simulink model "PPTS_pmsm"  (R2020b)
settings: Solver=ode3  StartTime=0.0  StopTime=10.0  FixedStep=0.0001  RelTol=0.0001
values from neighbouring files (symbols this model uses):
  a = 0.3    [initial_parameters_PPTS.m]
  a11 = 48    [initial_parameters_PPTS.m]
  a12 = 48    [initial_parameters_PPTS.m]
  a21 = 13    [initial_parameters_PPTS.m]
  a22 = 13    [initial_parameters_PPTS.m]
  B = 2e-3    (= 0.002)    [initial_parameters_PPTS.m]
  f = 1    [initial_parameters_PPTS.m]
  J = 8e-4    (= 0.0008)    [initial_parameters_PPTS.m]
  k1 = 240    [initial_parameters_PPTS.m]
  K1 = 220    [initial_parameters_PPTS.m]
  k2 = 240    [initial_parameters_PPTS.m]
  K2 = 220    [initial_parameters_PPTS.m]
  k3 = 240    [initial_parameters_PPTS.m]
  K3 = 220    [initial_parameters_PPTS.m]
  k4 = 240    [initial_parameters_PPTS.m]
  K4 = 220    [initial_parameters_PPTS.m]
  L = 0.1875    [initial_parameters_PPTS.m]
  n1 = 0.9    [initial_parameters_PPTS.m]
  n2 = 0.7    [initial_parameters_PPTS.m]
  P = 2    [initial_parameters_PPTS.m]
  psi_f = 0.945    [initial_parameters_PPTS.m]
  R = 12.5    [initial_parameters_PPTS.m]
  rh0 = 0.8    [initial_parameters_PPTS.m]
  rh0c = 0.9    [initial_parameters_PPTS.m]
  rho0 = 10.6    [initial_parameters_PPTS.m]
  rho01 = 0.6    [initial_parameters_PPTS.m]
  rho0c = 0.5    [initial_parameters_PPTS.m]
  rho0e = 0.6    [initial_parameters_PPTS.m]
  rhoTf = 0.1    [initial_parameters_PPTS.m]
  rhoTfc = 0.1    [initial_parameters_PPTS.m]
  rhoTfe = 0.1    [initial_parameters_PPTS.m]
  S = 2    [initial_parameters_PPTS.m]
  T = 0.1    [initial_parameters_PPTS.m]
  ta = 0.3    [initial_parameters_PPTS.m]
  Tf = 3    [initial_parameters_PPTS.m]
  Tfc = 3.8    [initial_parameters_PPTS.m]
  Tfe = 4    [initial_parameters_PPTS.m]
  th = 0.001    [initial_parameters_PPTS.m]
  v = 42.2    [initial_parameters_PPTS.m]
  v1 = 14    [initial_parameters_PPTS.m]
  v2 = 80    [initial_parameters_PPTS.m]
  v3 = 20    [initial_parameters_PPTS.m]
  X = 2    [initial_parameters_PPTS.m]
settings Model: Creator=Administrator  LastModifiedBy=62407

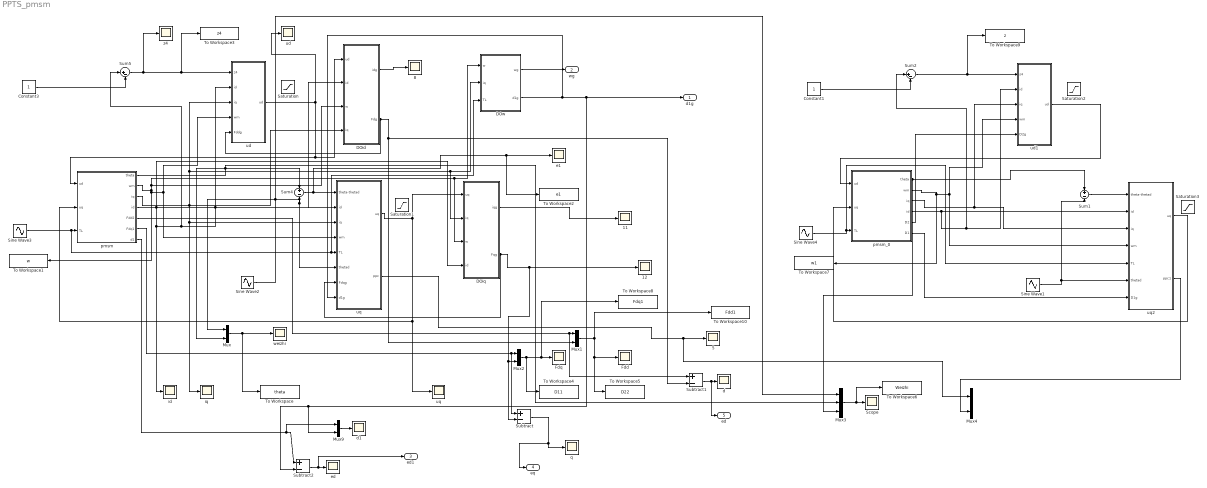
== system PPTS_pmsm ==
   {5,8,11..12} (4 alike) : Scope
  " Fdd" : Scope
  " Fdq" : Scope
  " d1 " : Scope
  " e1" : Scope
  " ed" : Scope
  " id" : Scope
  " iq" : Scope
  " ud" : Scope
  " uq" : Scope
  " z4" : Scope
  Constant1 : Constant
  Constant3 : Constant
  DOid : Subsystem
  DOiq : Subsystem
  DOw : Subsystem
  Mux{,1..2,4,9} (5 alike) : Mux  Inputs=2
  Mux3 : Mux  Inputs=3
  Saturation{,1..3} (4 alike) : Saturate  UpperLimit=120  LowerLimit=-120
  Scope : Scope
  Sine Wave1 : Sin  Amplitude=1.2  Frequency=1.8*pi  SampleTime=0
  Sine Wave2 : Sin  Amplitude=1.2  Frequency=1.8*pi  SampleTime=0
  Sine Wave3 : Sin  Amplitude=0.8  Frequency=0.5*pi  SampleTime=0
  Sine Wave4 : Sin  Amplitude=0.8  Frequency=0.5*pi  SampleTime=0
  Subtract : Sum  Inputs=+-
  Subtract1 : Sum  Inputs=+-
  Subtract2 : Sum  Inputs=+-
  Sum1 : Sum  Inputs=+|-
  Sum2 : Sum  Inputs=|+-
  Sum4 : Sum  Inputs=+|-
  Sum5 : Sum  Inputs=|+-
  To Workspace : ToWorkspace  VariableName=theta  SaveFormat=Timeseries  SampleTime=-1
  To Workspace1 : ToWorkspace  VariableName=w  SaveFormat=Timeseries  SampleTime=-1
  To Workspace10 : ToWorkspace  VariableName=Fdd1  SaveFormat=Timeseries  SampleTime=-1
  To Workspace2 : ToWorkspace  VariableName=e1  SaveFormat=Timeseries  SampleTime=-1
  To Workspace3 : ToWorkspace  VariableName=z4  SaveFormat=Timeseries  SampleTime=-1
  To Workspace4 : ToWorkspace  VariableName=D11  SaveFormat=Timeseries  SampleTime=-1
  To Workspace5 : ToWorkspace  VariableName=D22  SaveFormat=Timeseries  SampleTime=-1
  To Workspace6 : ToWorkspace  VariableName=Weizhi  SaveFormat=Timeseries  SampleTime=-1
  To Workspace7 : ToWorkspace  VariableName=w1  SaveFormat=Timeseries  SampleTime=-1
  To Workspace8 : ToWorkspace  VariableName=Fdq1  SaveFormat=Timeseries  SampleTime=-1
  To Workspace9 : ToWorkspace  VariableName=z  SaveFormat=Timeseries  SampleTime=-1
  d : Scope
  pmsm : Subsystem
  pmsm_0 : Subsystem
  q : Scope
  ud : Subsystem
  ud1 : Subsystem
  uq : Subsystem
  uq2 : Subsystem
  weizhi : Scope
  d1g : Outport
  wg : Outport  Port=2
  ed1 : Outport  Port=3
  eq : Outport  Port=4
  ed : Outport  Port=5
  wires:
  DOw/2(d1g) -> uq/8(d1g), Subtract2/2, Mux9/2, d1g/1
  Subtract1/1 -> ed/1, d/1
  uq/2(ppc) -> Mux4/1, " 5"/1
  Subtract2/1 -> ed1/1, " ed"/1
  Subtract/1 -> eq/1, q/1
  pmsm/4(id) -> DOiq/4(id), " id"/1, Sum5/1, ud/2(id), uq/2(id), DOid/2(" id")
  DOw/1(wg) -> wg/1
  pmsm/5(Fdd2) -> Subtract1/1, Mux1/1
  Sine Wave3/1 -> DOw/3(TL), uq/5(TL), pmsm/3(TL)
  pmsm/6(Fdq1) -> Subtract/1, Mux2/1
  pmsm/7(d1) -> Mux9/1, Subtract2/1
  Mux9/1 -> " d1 "/1
  Sum5/1 -> ud/1(z4), To Workspace3/1, " z4"/1
  Mux2/1 -> To Workspace4/1, To Workspace8/1, " Fdq"/1
  pmsm/2(wm) -> DOiq/3(w), DOw/1(w), DOid/3(w), uq/4(wm), ud/4(wm), To Workspace1/1
  Sum4/1 -> uq/1(theta-thetad), To Workspace2/1, " e1"/1
  Mux1/1 -> To Workspace10/1, To Workspace5/1, " Fdd"/1
  DOiq/2(Fqg) -> uq/7(Fdqg), Subtract/2, Mux2/2, " 12"/1
  DOiq/1(iqg) -> " 11"/1
  Mux/1 -> To Workspace/1, weizhi/1
  pmsm/1(theta) -> Mux3/2, Mux/2, Sum4/1
  Sine Wave2/1 -> Mux3/1, uq/6(thetad), Sum4/2, Mux/1
  Constant3/1 -> Sum5/2
  pmsm/3(iq) -> DOw/2(iq), DOiq/2(iq), ud/3(iq), uq/3(iq), " iq"/1, DOid/4(iq)
  DOid/1(idg) -> " 8"/1
  DOid/2(Fdg) -> ud/5(Fddg), Subtract1/2, Mux1/2
  uq/1(uq) -> DOiq/1(uq), pmsm/2(uq), " uq"/1
  ud/1(ud) -> pmsm/1(ud), DOid/1(ud), " ud"/1
  pmsm_0/2(wm) -> uq2/4(wm), ud1/4(wm), To Workspace7/1
  Sum2/1 -> ud1/1(s4), To Workspace9/1
  ud1/1(ud) -> pmsm_0/1(ud)
  pmsm_0/5(D2) -> ud1/5(D2g)
  pmsm_0/3(iq) -> ud1/3(iq), uq2/3(iq)
  Sine Wave1/1 -> uq2/6(thetad), Sum1/2
  Constant1/1 -> Sum2/2
  pmsm_0/1(theta) -> Mux3/3, Sum1/1
  Sum1/1 -> uq2/1(theta-thetad)
  pmsm_0/4(id) -> uq2/2(id), Sum2/1, ud1/2(id)
  Sine Wave4/1 -> uq2/5(TL), pmsm_0/3(TL)
  uq2/1(uq) -> pmsm_0/2(uq)
  pmsm_0/6(D1) -> uq2/7(D1g)
  Mux3/1 -> To Workspace6/1, Scope/1
  uq2/2(ppc1) -> Mux4/2

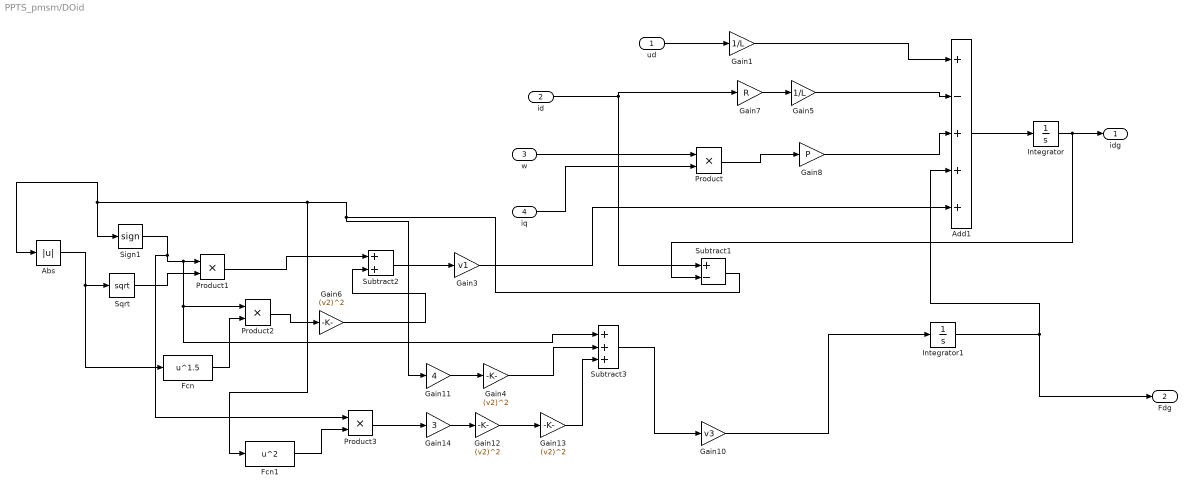
== system PPTS_pmsm/DOid ==
  ud : Inport
  " id" : Inport  Port=2
  w : Inport  Port=3
  iq : Inport  Port=4
  Abs : Abs
  Add1 : Sum  Inputs=+-+++
  Fcn : Fcn  Expr=u^1.5
  Fcn1 : Fcn  Expr=u^2
  Gain1 : Gain  Gain=1/L
  Gain10 : Gain  Gain=v3
  Gain11 : Gain  Gain=4
  Gain{4,6,12..13} (4 alike) : Gain  Gain=(v2)^2
  Gain14 : Gain  Gain=3
  Gain3 : Gain  Gain=v1
  Gain5 : Gain  Gain=1/L
  Gain7 : Gain  Gain=R
  Gain8 : Gain  Gain=P
  Integrator : Integrator
  Integrator1 : Integrator
  Product{,1..3} (4 alike) : Product
  Sign1 : Signum
  Sqrt : Sqrt  SaturateOnIntegerOverflow=on
  Subtract1 : Sum  Inputs=+-
  Subtract2 : Sum
  Subtract3 : Sum  Inputs=+++
  idg : Outport
  Fdg : Outport  Port=2
  wires:
  iq/1 -> Product/2
  w/1 -> Product/1
  Product/1 -> Gain8/1
  Gain8/1 -> Add1/3
  Gain5/1 -> Add1/2
  Integrator/1 -> Subtract1/2, idg/1
  Gain7/1 -> Gain5/1
  ud/1 -> Gain1/1
  Add1/1 -> Integrator/1
  Gain1/1 -> Add1/1
  Integrator1/1 -> Fdg/1, Add1/4
  " id"/1 -> Subtract1/1, Gain7/1
  Gain6/1 -> Subtract2/2
  Gain11/1 -> Gain4/1
  Product2/1 -> Gain6/1
  Gain13/1 -> Subtract3/3
  Subtract2/1 -> Gain3/1
  Fcn/1 -> Product2/2
  Subtract1/1 -> Fcn1/1, Abs/1, Sign1/1, Gain11/1
  Sqrt/1 -> Product1/2
  Fcn1/1 -> Product3/2
  Gain4/1 -> Subtract3/2
  Abs/1 -> Fcn/1, Sqrt/1
  Product1/1 -> Subtract2/1
  Gain12/1 -> Gain13/1
  Subtract3/1 -> Gain10/1
  Product3/1 -> Gain14/1
  Gain14/1 -> Gain12/1
  Sign1/1 -> Product2/1, Subtract3/1, Product1/1, Product3/1
  Gain10/1 -> Integrator1/1
  Gain3/1 -> Add1/5

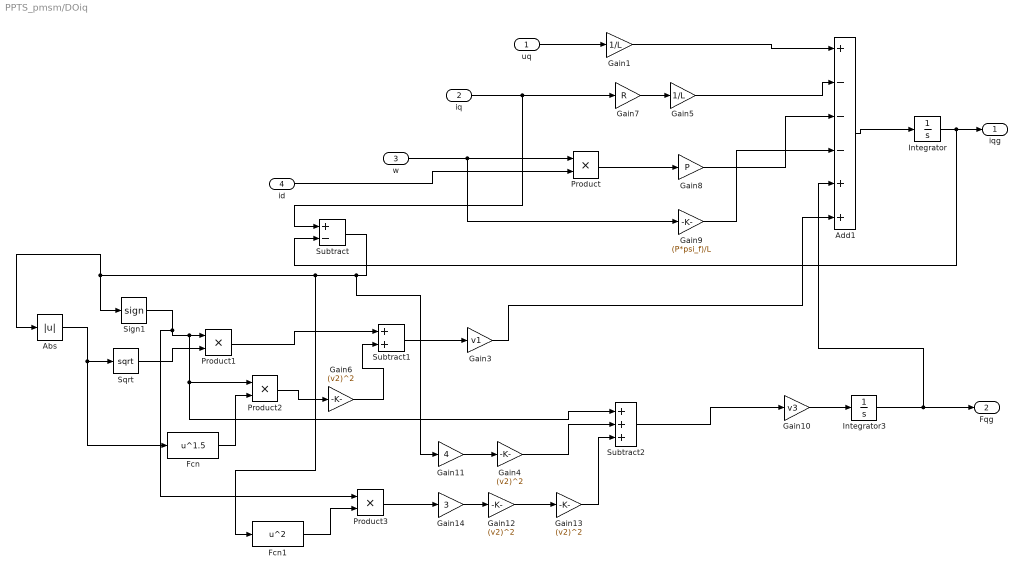
== system PPTS_pmsm/DOiq ==
  uq : Inport
  iq : Inport  Port=2
  w : Inport  Port=3
  id : Inport  Port=4
  Abs : Abs
  Add1 : Sum  Inputs=+---++
  Fcn : Fcn  Expr=u^1.5
  Fcn1 : Fcn  Expr=u^2
  Gain1 : Gain  Gain=1/L
  Gain10 : Gain  Gain=v3
  Gain11 : Gain  Gain=4
  Gain{4,6,12..13} (4 alike) : Gain  Gain=(v2)^2
  Gain14 : Gain  Gain=3
  Gain3 : Gain  Gain=v1
  Gain5 : Gain  Gain=1/L
  Gain7 : Gain  Gain=R
  Gain8 : Gain  Gain=P
  Gain9 : Gain  Gain=(P*psi_f)/L
  Integrator : Integrator
  Integrator3 : Integrator
  Product{,1..3} (4 alike) : Product
  Sign1 : Signum
  Sqrt : Sqrt  SaturateOnIntegerOverflow=on
  Subtract : Sum  Inputs=+-
  Subtract1 : Sum
  Subtract2 : Sum  Inputs=+++
  iqg : Outport
  Fqg : Outport  Port=2
  wires:
  Add1/1 -> Integrator/1
  uq/1 -> Gain1/1
  Gain7/1 -> Gain5/1
  Integrator/1 -> Subtract/2, iqg/1
  Gain5/1 -> Add1/2
  Gain8/1 -> Add1/3
  Product/1 -> Gain8/1
  w/1 -> Gain9/1, Product/1
  id/1 -> Product/2
  Gain9/1 -> Add1/4
  Gain1/1 -> Add1/1
  Integrator3/1 -> Fqg/1, Add1/5
  iq/1 -> Gain7/1, Subtract/1
  Sign1/1 -> Product2/1, Subtract2/1, Product1/1, Product3/1
  Sqrt/1 -> Product1/2
  Abs/1 -> Fcn/1, Sqrt/1
  Subtract/1 -> Gain11/1, Fcn1/1, Abs/1, Sign1/1
  Product1/1 -> Subtract1/1
  Fcn/1 -> Product2/2
  Product2/1 -> Gain6/1
  Gain6/1 -> Subtract1/2
  Subtract1/1 -> Gain3/1
  Gain3/1 -> Add1/6
  Gain10/1 -> Integrator3/1
  Gain11/1 -> Gain4/1
  Gain4/1 -> Subtract2/2
  Gain12/1 -> Gain13/1
  Gain14/1 -> Gain12/1
  Gain13/1 -> Subtract2/3
  Product3/1 -> Gain14/1
  Fcn1/1 -> Product3/2
  Subtract2/1 -> Gain10/1

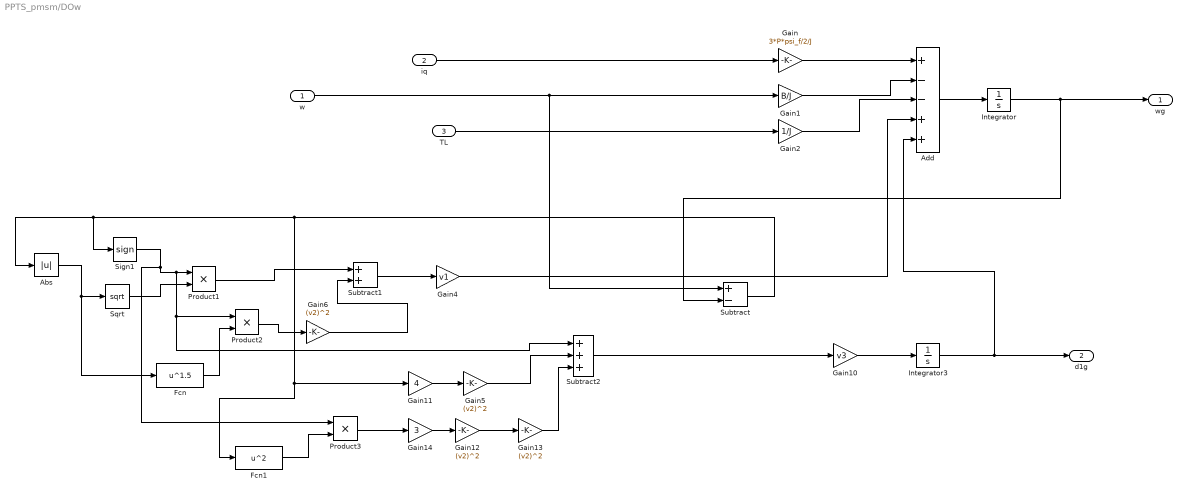
== system PPTS_pmsm/DOw ==
  w : Inport
  iq : Inport  Port=2
  TL : Inport  Port=3
  Abs : Abs
  Add : Sum  Inputs=+--++
  Fcn : Fcn  Expr=u^1.5
  Fcn1 : Fcn  Expr=u^2
  Gain : Gain  Gain=3*P*psi_f/2/J
  Gain1 : Gain  Gain=B/J
  Gain10 : Gain  Gain=v3
  Gain11 : Gain  Gain=4
  Gain{5..6,12..13} (4 alike) : Gain  Gain=(v2)^2
  Gain14 : Gain  Gain=3
  Gain2 : Gain  Gain=1/J
  Gain4 : Gain  Gain=v1
  Integrator : Integrator
  Integrator3 : Integrator
  Product1 : Product
  Product2 : Product
  Product3 : Product
  Sign1 : Signum
  Sqrt : Sqrt  SaturateOnIntegerOverflow=on
  Subtract : Sum  Inputs=+-
  Subtract1 : Sum
  Subtract2 : Sum  Inputs=+++
  wg : Outport
  d1g : Outport  Port=2
  wires:
  TL/1 -> Gain2/1
  Add/1 -> Integrator/1
  Integrator/1 -> wg/1, Subtract/2
  Gain2/1 -> Add/3
  Gain1/1 -> Add/2
  Gain10/1 -> Integrator3/1
  Gain/1 -> Add/1
  iq/1 -> Gain/1
  w/1 -> Subtract/1, Gain1/1
  Gain6/1 -> Subtract1/2
  Gain11/1 -> Gain5/1
  Product2/1 -> Gain6/1
  Gain13/1 -> Subtract2/3
  Subtract1/1 -> Gain4/1
  Fcn/1 -> Product2/2
  Sqrt/1 -> Product1/2
  Fcn1/1 -> Product3/2
  Gain5/1 -> Subtract2/2
  Abs/1 -> Fcn/1, Sqrt/1
  Product1/1 -> Subtract1/1
  Gain12/1 -> Gain13/1
  Subtract2/1 -> Gain10/1
  Product3/1 -> Gain14/1
  Gain14/1 -> Gain12/1
  Sign1/1 -> Product2/1, Subtract2/1, Product1/1, Product3/1
  Subtract/1 -> Fcn1/1, Gain11/1, Abs/1, Sign1/1
  Integrator3/1 -> Add/5, d1g/1
  Gain4/1 -> Add/4

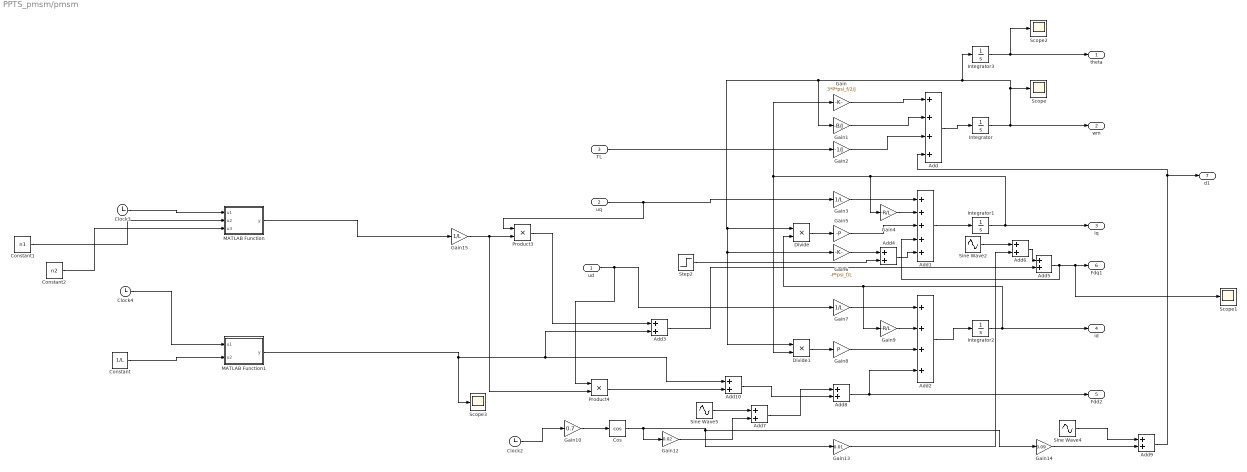
== system PPTS_pmsm/pmsm ==
  ud : Inport
  uq : Inport  Port=2
  TL : Inport  Port=3
  Add : Sum  Inputs=++++
  Add1 : Sum  Inputs=+++++
  Add{3..10} (8 alike) : Sum
  Add2 : Sum  Inputs=++++
  Clock2 : Clock
  Clock3 : Clock
  Clock4 : Clock
  Constant : Constant  Value=1/L
  Constant1 : Constant  Value=n1
  Constant2 : Constant  Value=n2
  Cos : Trigonometry  Operator=cos
  Divide : Product  Inputs=**
  Divide1 : Product  Inputs=**
  Gain : Gain  Gain=3*P*psi_f/2/J
  Gain1 : Gain  Gain=-B/J
  Gain10 : Gain  Gain=0.7
  Gain12 : Gain  Gain=0.02
  Gain13 : Gain  Gain=0.01
  Gain14 : Gain  Gain=0.09
  Gain15 : Gain  Gain=1/L
  Gain2 : Gain  Gain=-1/J
  Gain3 : Gain  Gain=1/L
  Gain4 : Gain  Gain=-R/L
  Gain5 : Gain  Gain=-P
  Gain6 : Gain  Gain=-P*psi_f/L
  Gain7 : Gain  Gain=1/L
  Gain8 : Gain  Gain=P
  Gain9 : Gain  Gain=-R/L
  Integrator : Integrator
  Integrator1 : Integrator
  Integrator2 : Integrator
  Integrator3 : Integrator  InitialCondition=0.1
  MATLAB Function : MATLAB Function  TreatAsAtomicUnit=on
  MATLAB Function1 : MATLAB Function  TreatAsAtomicUnit=on
  Product3 : Product
  Product4 : Product
  Scope{,1..3} (4 alike) : Scope
  Sine Wave2 : Sin  Amplitude=0.03  Frequency=1.6  SampleTime=0
  Sine Wave4 : Sin  Amplitude=0.04  Frequency=1.6  SampleTime=0
  Sine Wave5 : Sin  Amplitude=0.08  Frequency=1.6  SampleTime=0
  Step2 : Step  Time=6  After=0  SampleTime=0
  theta : Outport
  wm : Outport  Port=2
  iq : Outport  Port=3
  id : Outport  Port=4
  Fdd2 : Outport  Port=5
  Fdq1 : Outport  Port=6
  d1 : Outport  Port=7
  wires:
  Add/1 -> Integrator/1
  Add1/1 -> Integrator1/1
  Gain/1 -> Add/1
  Gain1/1 -> Add/2
  TL/1 -> Gain2/1
  Gain3/1 -> Add1/1
  Gain4/1 -> Add1/2
  Gain5/1 -> Add1/3
  Divide/1 -> Gain5/1
  Add2/1 -> Integrator2/1
  Gain7/1 -> Add2/1
  Divide1/1 -> Gain8/1
  Gain9/1 -> Add2/2
  Integrator1/1 -> iq/1, Divide1/2, Gain/1, Gain4/1
  Integrator2/1 -> id/1, Gain9/1, Divide/2
  Gain2/1 -> Add/3
  Gain8/1 -> Add2/3
  Integrator/1 -> wm/1, Scope/1, Integrator3/1, Divide/1, Gain6/1, Divide1/1, Gain1/1
  Gain6/1 -> Add4/1
  Step2/1 -> Add4/2
  uq/1 -> Product3/1, Gain3/1
  ud/1 -> Product4/1, Gain7/1
  Add5/1 -> Add1/4, Scope1/1, Fdq1/1
  Add8/1 -> Fdd2/1, Add2/4
  Integrator3/1 -> theta/1, Scope2/1
  Add4/1 -> Add1/5
  Add6/1 -> Add5/1
  Sine Wave2/1 -> Add6/1
  Sine Wave5/1 -> Add7/1
  Add7/1 -> Add8/1
  Gain10/1 -> Cos/1
  Cos/1 -> Gain14/1, Gain13/1, Gain12/1
  Gain12/1 -> Add7/2
  Gain13/1 -> Add6/2
  Add9/1 -> d1/1, Add/4
  Clock2/1 -> Gain10/1
  Gain14/1 -> Add9/2
  Sine Wave4/1 -> Add9/1
  MATLAB Function1/1(y) -> Scope3/1, Add10/1, Add3/2
  Add3/1 -> Add5/2
  MATLAB Function/1(y) -> Gain15/1
  Gain15/1 -> Product4/2, Product3/2
  Add10/1 -> Add8/2
  Product3/1 -> Add3/1
  Product4/1 -> Add10/2
  Clock3/1 -> MATLAB Function/1(u1)
  Clock4/1 -> MATLAB Function1/1(u1)
  Constant/1 -> MATLAB Function1/2(u2)
  Constant1/1 -> MATLAB Function/2(u2)
  Constant2/1 -> MATLAB Function/3(u3)

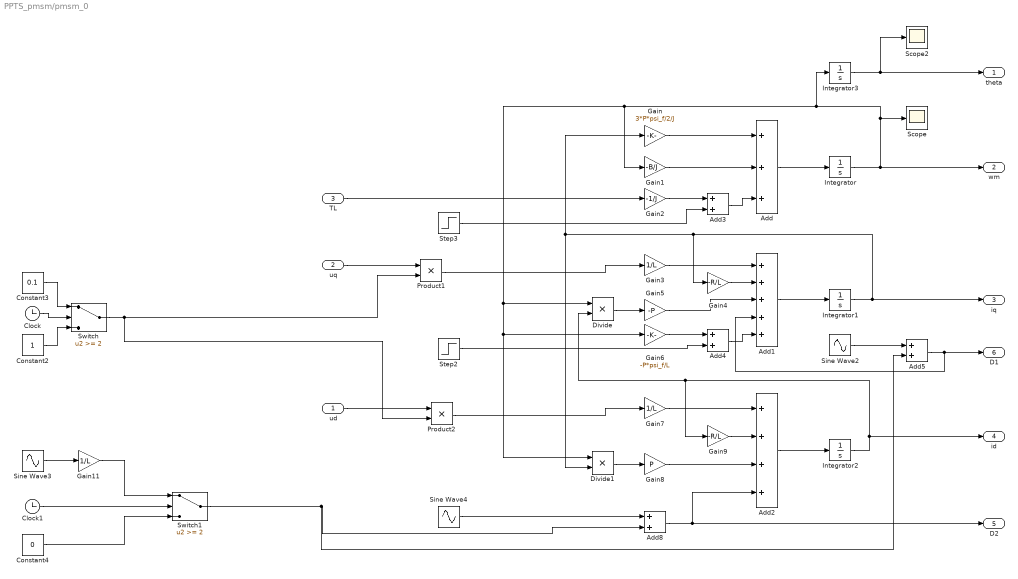
== system PPTS_pmsm/pmsm_0 ==
  ud : Inport
  uq : Inport  Port=2
  TL : Inport  Port=3
  Add : Sum  Inputs=+++
  Add1 : Sum  Inputs=+++++
  Add2 : Sum  Inputs=++++
  Add{3..5,8} (4 alike) : Sum
  Clock : Clock
  Clock1 : Clock
  Constant2 : Constant
  Constant3 : Constant  Value=0.1
  Constant4 : Constant  Value=0
  Divide : Product  Inputs=**
  Divide1 : Product  Inputs=**
  Gain : Gain  Gain=3*P*psi_f/2/J
  Gain1 : Gain  Gain=-B/J
  Gain11 : Gain  Gain=1/L
  Gain2 : Gain  Gain=-1/J
  Gain3 : Gain  Gain=1/L
  Gain4 : Gain  Gain=-R/L
  Gain5 : Gain  Gain=-P
  Gain6 : Gain  Gain=-P*psi_f/L
  Gain7 : Gain  Gain=1/L
  Gain8 : Gain  Gain=P
  Gain9 : Gain  Gain=-R/L
  Integrator : Integrator
  Integrator1 : Integrator
  Integrator2 : Integrator
  Integrator3 : Integrator  InitialCondition=0.1
  Product1 : Product
  Product2 : Product
  Scope : Scope
  Scope2 : Scope
  Sine Wave2 : Sin  Amplitude=5.1  Frequency=3*pi  Phase=9.8  SampleTime=0
  Sine Wave3 : Sin  Amplitude=2.5  Frequency=2*pi  SampleTime=0
  Sine Wave4 : Sin  Amplitude=3.5  Frequency=6.9  Phase=3.2  SampleTime=0
  Step2 : Step  Time=6  After=0  SampleTime=0
  Step3 : Step  Time=6  After=0  SampleTime=0
  Switch : Switch  Threshold=2
  Switch1 : Switch  Threshold=2
  theta : Outport
  wm : Outport  Port=2
  iq : Outport  Port=3
  id : Outport  Port=4
  D2 : Outport  Port=5
  D1 : Outport  Port=6
  wires:
  Add/1 -> Integrator/1
  Add1/1 -> Integrator1/1
  Gain/1 -> Add/1
  Gain1/1 -> Add/2
  TL/1 -> Gain2/1
  Gain3/1 -> Add1/1
  Gain4/1 -> Add1/2
  Gain5/1 -> Add1/3
  Divide/1 -> Gain5/1
  Add2/1 -> Integrator2/1
  Gain7/1 -> Add2/1
  Divide1/1 -> Gain8/1
  Gain9/1 -> Add2/2
  Integrator1/1 -> iq/1, Divide1/2, Gain/1, Gain4/1
  Integrator2/1 -> id/1, Gain9/1, Divide/2
  Gain2/1 -> Add3/1
  Add3/1 -> Add/3
  Step3/1 -> Add3/2
  Gain8/1 -> Add2/3
  Integrator/1 -> wm/1, Scope/1, Integrator3/1, Divide/1, Gain6/1, Divide1/1, Gain1/1
  Gain6/1 -> Add4/1
  Step2/1 -> Add4/2
  Sine Wave4/1 -> Add8/1
  Sine Wave2/1 -> Add5/1
  uq/1 -> Product1/1
  Add5/1 -> Add1/4, D1/1
  Add8/1 -> D2/1, Add2/4
  Clock/1 -> Switch/2
  Constant2/1 -> Switch/3
  Integrator3/1 -> theta/1, Scope2/1
  Constant3/1 -> Switch/1
  Clock1/1 -> Switch1/2
  Constant4/1 -> Switch1/3
  Gain11/1 -> Switch1/1
  Add4/1 -> Add1/5
  Sine Wave3/1 -> Gain11/1
  Switch/1 -> Product1/2, Product2/2
  Product1/1 -> Gain3/1
  ud/1 -> Product2/1
  Product2/1 -> Gain7/1
  Switch1/1 -> Add5/2, Add8/2

== system PPTS_pmsm/ud ==
  z4 : Inport
  id : Inport  Port=2
  iq : Inport  Port=3
  wm : Inport  Port=4
  Fddg : Inport  Port=5
  Abs : Abs
  Add1 : Sum  Inputs=--+--
  Derivative : Derivative
  Fcn : Fcn  Expr=1/u
  Gain1 : Gain  Gain=L
  Gain2 : Gain  Gain=k4
  Gain3 : Gain  Gain=2
  Gain4 : Gain  Gain=R
  Gain5 : Gain  Gain=1/L
  Gain6 : Gain  Gain=P
  Product1 : Product
  Product2 : Product
  Product3 : Product
  chiduhanshu : Subsystem
  ud : Outport
  wires:
  wm/1 -> Product2/2
  iq/1 -> Product2/1
  Product2/1 -> Gain6/1
  Gain6/1 -> Add1/4
  Gain5/1 -> Add1/3
  Gain4/1 -> Gain5/1
  id/1 -> Gain4/1
  Gain3/1 -> Product1/1
  Product1/1 -> Add1/2
  Add1/1 -> Gain1/1
  Gain1/1 -> ud/1
  Gain2/1 -> Add1/1
  z4/1 -> Gain3/1, Gain2/1
  Fddg/1 -> Add1/5
  Product3/1 -> Product1/2
  chiduhanshu/1(Out1) -> Derivative/1, Fcn/1
  Fcn/1 -> Product3/2
  Derivative/1 -> Abs/1
  Abs/1 -> Product3/1

== system PPTS_pmsm/ud1 ==
  s4 : Inport
  id : Inport  Port=2
  iq : Inport  Port=3
  wm : Inport  Port=4
  D2g : Inport  Port=5
  Add1 : Sum  Inputs=-+--
  Gain1 : Gain  Gain=L
  Gain2 : Gain  Gain=K4
  Gain4 : Gain  Gain=R
  Gain5 : Gain  Gain=1/L
  Gain6 : Gain  Gain=P
  Product2 : Product
  ud : Outport
  wires:
  wm/1 -> Product2/2
  iq/1 -> Product2/1
  Product2/1 -> Gain6/1
  Gain4/1 -> Gain5/1
  id/1 -> Gain4/1
  Add1/1 -> Gain1/1
  Gain1/1 -> ud/1
  D2g/1 -> Add1/4
  s4/1 -> Gain2/1
  Gain5/1 -> Add1/2
  Gain6/1 -> Add1/3
  Gain2/1 -> Add1/1

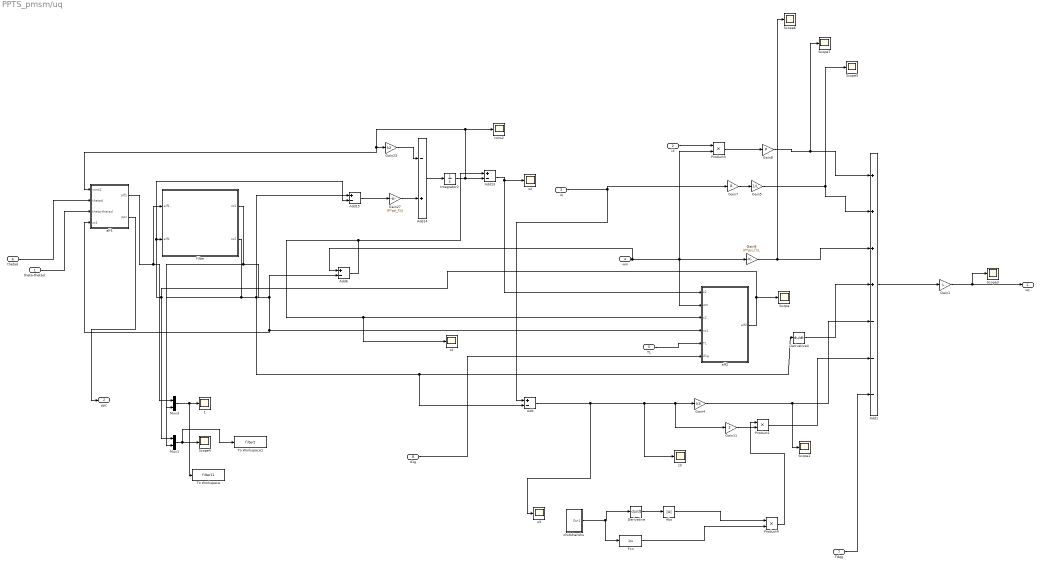
== system PPTS_pmsm/uq ==
  theta-thetad : Inport
  id : Inport  Port=2
  iq : Inport  Port=3
  wm : Inport  Port=4
  TL : Inport  Port=5
  thetad : Inport  Port=6
  Fdqg : Inport  Port=7
  d1g : Inport  Port=8
  1 : Scope
  Abs : Abs
  Add{,6,13,15} (4 alike) : Sum  Inputs=+-
  Add1 : Sum  Inputs=++++---
  Add14 : Sum  Inputs=-+
  Derivative : Derivative
  Derivative4 : Derivative
  Fcn : Fcn  Expr=1/u
  Gain1 : Gain  Gain=L
  Gain11 : Gain  Gain=2
  Gain23 : Gain  Gain=k2
  Gain27 : Gain  Gain=(P*psi_f)/J
  Gain4 : Gain  Gain=k3
  Gain5 : Gain  Gain=1/L
  Gain7 : Gain  Gain=R
  Gain8 : Gain  Gain=P
  Gain9 : Gain  Gain=(P*psi_f)/L
  Integrator2 : Integrator
  Mux1 : Mux  Inputs=2
  Mux3 : Mux  Inputs=2
  Product1 : Product
  Product3 : Product
  Product4 : Product
  Scope{,1,3..7} (7 alike) : Scope
  To Workspace : ToWorkspace  VariableName=filter11  SaveFormat=Timeseries  SampleTime=-1
  To Workspace1 : ToWorkspace  VariableName=filter2  SaveFormat=Timeseries  SampleTime=-1
  alf1 : Subsystem
  alf2 : Subsystem
  chiduhanshu : Subsystem
  cons2 : Scope
  filter : Subsystem
  s2 : Scope
  s3 : Scope
  z2 : Scope
  z3 : Scope
  uq : Outport
  ppc : Outport  Port=2
  wires:
  Gain9/1 -> Scope6/1, Add1/3
  Gain7/1 -> Gain5/1
  Gain8/1 -> Scope7/1, Add1/1
  Product3/1 -> Gain8/1
  wm/1 -> Gain9/1, Product3/2, alf2/2(wm), Add6/1
  id/1 -> Product3/1
  iq/1 -> Gain7/1, Add/1
  Gain5/1 -> Add1/2, Scope5/1
  Derivative4/1 -> Add1/4
  Add/1 -> s3/1, Gain11/1, Gain4/1, z3/1
  Gain11/1 -> Product1/2
  Gain4/1 -> Scope1/1, Add1/5
  Product1/1 -> Add1/6
  filter/1(xc1) -> alf1/4(xc1), alf2/4(xc1), Add6/2, Mux3/2
  Fdqg/1 -> Add1/7
  Add13/1 -> alf2/1(s2), s2/1
  TL/1 -> alf2/5(TL)
  Integrator2/1 -> cons2/1, alf1/1(cons2), Gain23/1, Add13/2
  thetad/1 -> alf1/2(thetad)
  theta-thetad/1 -> alf1/3(theta-thetad)
  alf1/1(alf1) -> Mux3/1, filter/1(alf1)
  Mux3/1 -> To Workspace/1, 1/1
  Mux1/1 -> To Workspace1/1, Scope4/1
  Gain1/1 -> uq/1, Scope3/1
  alf1/2(ppc) -> ppc/1
  filter/2(xc2) -> Add15/1, Add/2, Derivative4/1, Mux1/2
  Gain27/1 -> Add14/2
  Add14/1 -> Integrator2/1
  Add6/1 -> Add13/1, z2/1, alf2/3(z2)
  Gain23/1 -> Add14/1
  alf2/1(alf2) -> Add15/2, filter/2(alf2), Mux1/1, Scope/1
  Add15/1 -> Gain27/1
  Product4/1 -> Product1/1
  d1g/1 -> alf2/6(d1g)
  Add1/1 -> Gain1/1
  chiduhanshu/1(Out1) -> Fcn/1, Derivative/1
  Derivative/1 -> Abs/1
  Abs/1 -> Product4/1
  Fcn/1 -> Product4/2

== system PPTS_pmsm/uq2 ==
  theta-thetad : Inport
  id : Inport  Port=2
  iq : Inport  Port=3
  wm : Inport  Port=4
  TL : Inport  Port=5
  thetad : Inport  Port=6
  D1g : Inport  Port=7
  Add : Sum  Inputs=+-
  Add1 : Sum  Inputs=+++-+-
  Add2 : Sum  Inputs=+-
  Derivative : Derivative
  Gain1 : Gain  Gain=L
  Gain4 : Gain  Gain=K3
  Gain5 : Gain  Gain=1/L
  Gain7 : Gain  Gain=R
  Gain8 : Gain  Gain=P
  Gain9 : Gain  Gain=(P*psi_f)/L
  Product3 : Product
  Scope{3,5..7} (4 alike) : Scope
  alf1 : Subsystem
  alf2 : Subsystem
  uq : Outport
  ppc1 : Outport  Port=2
  wires:
  Gain9/1 -> Scope6/1, Add1/3
  Gain7/1 -> Gain5/1
  Gain8/1 -> Scope7/1, Add1/1
  Product3/1 -> Gain8/1
  wm/1 -> alf2/2(wm), Add/1, Product3/2, Gain9/1
  id/1 -> Product3/1
  iq/1 -> Add2/1, Gain7/1
  Add1/1 -> Gain1/1
  Gain5/1 -> Scope5/1, Add1/2
  thetad/1 -> alf1/1(thetad)
  theta-thetad/1 -> alf1/2(theta-thetad)
  Gain1/1 -> uq/1, Scope3/1
  D1g/1 -> Add1/6
  alf1/1(alf1) -> alf2/3(alf1), Add/2
  TL/1 -> alf2/4(TL)
  Add/1 -> alf2/1(s2)
  Derivative/1 -> Add1/5
  alf2/1(alf2) -> Add2/2, Derivative/1
  Gain4/1 -> Add1/4
  Add2/1 -> Gain4/1
  alf1/2(ppc) -> ppc1/1

== system PPTS_pmsm/ud/chiduhanshu ==
  Clock : Clock
  Clock1 : Clock
  Constant1 : Constant  Value=T
  Constant{2,4..6} (4 alike) : Constant
  Constant3 : Constant  Value=T
  Constant7 : Constant  Value=T
  Constant8 : Constant  Value=1/T
  Exp : Math  SaturateOnIntegerOverflow=on
  Fcn : Fcn  Expr=u^3
  Gain7 : Gain  Gain=a
  Gain8 : Gain  Gain=a
  Product : Product
  Subtract{1..6} (6 alike) : Sum  Inputs=+-
  Switch : Switch  Threshold=T
  Switch1 : Switch  Threshold=T
  Tanh : Trigonometry  Operator=tanh
  Out1 : Outport
  wires:
  Subtract5/1 -> Switch/3
  Gain7/1 -> Tanh/1
  Subtract4/1 -> Gain8/1
  Gain8/1 -> Exp/1
  Clock/1 -> Subtract4/2, Switch/2, Subtract2/1
  Exp/1 -> Subtract5/1
  Constant1/1 -> Subtract2/2
  Constant2/1 -> Subtract3/1
  Subtract2/1 -> Gain7/1
  Subtract3/1 -> Switch/1
  Tanh/1 -> Subtract3/2
  Constant3/1 -> Subtract4/1
  Constant4/1 -> Subtract5/2
  Constant5/1 -> Switch1/1
  Clock1/1 -> Subtract6/2, Switch1/2
  Constant6/1 -> Subtract1/1
  Constant7/1 -> Subtract6/1
  Subtract6/1 -> Product/1
  Constant8/1 -> Product/2
  Product/1 -> Fcn/1
  Fcn/1 -> Subtract1/2
  Subtract1/1 -> Switch1/3
  Switch/1 -> Out1/1

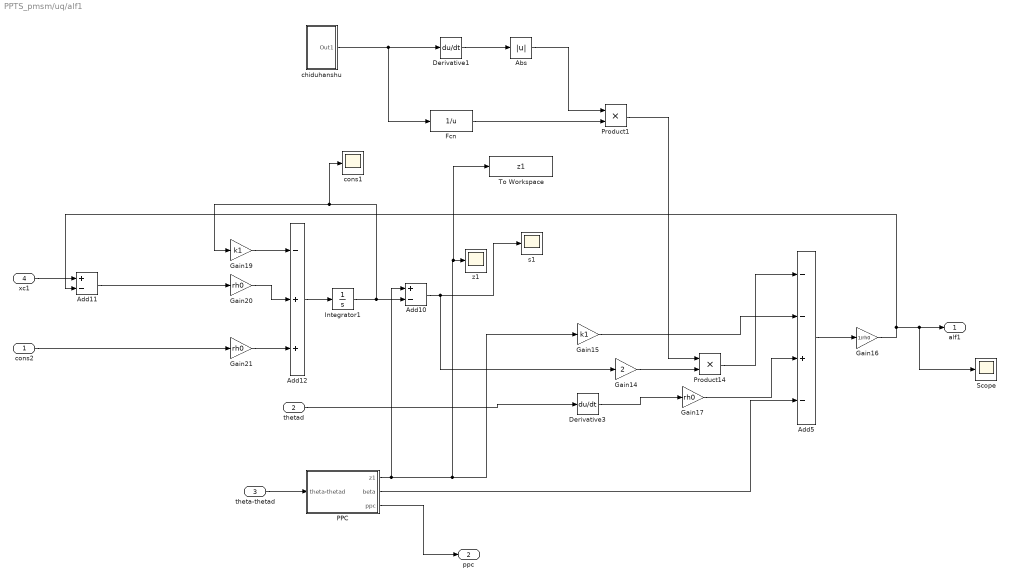
== system PPTS_pmsm/uq/alf1 ==
  cons2 : Inport
  thetad : Inport  Port=2
  theta-thetad : Inport  Port=3
  xc1 : Inport  Port=4
  Abs : Abs
  Add10 : Sum  Inputs=+-
  Add11 : Sum  Inputs=+-
  Add12 : Sum  Inputs=-++
  Add5 : Sum  Inputs=--+-
  Derivative1 : Derivative
  Derivative3 : Derivative
  Fcn : Fcn  Expr=1/u
  Gain14 : Gain  Gain=2
  Gain15 : Gain  Gain=k1
  Gain16 : Gain  Gain=1/rh0
  Gain17 : Gain  Gain=rh0
  Gain19 : Gain  Gain=k1
  Gain20 : Gain  Gain=rh0
  Gain21 : Gain  Gain=rh0
  Integrator1 : Integrator
  PPC : Subsystem
  Product1 : Product
  Product14 : Product
  Scope : Scope
  To Workspace : ToWorkspace  VariableName=z1  SaveFormat=Timeseries  SampleTime=-1
  chiduhanshu : Subsystem
  cons1 : Scope
  s1 : Scope
  z1 : Scope
  alf1 : Outport
  ppc : Outport  Port=2
  wires:
  theta-thetad/1 -> PPC/1(theta-thetad)
  Add5/1 -> Gain16/1
  PPC/2(beta) -> Add5/4
  Gain17/1 -> Add5/3
  Product14/1 -> Add5/1
  Gain15/1 -> Add5/2
  PPC/3(ppc) -> ppc/1
  cons2/1 -> Gain21/1
  Gain21/1 -> Add12/3
  Add10/1 -> Gain14/1, s1/1
  thetad/1 -> Derivative3/1
  Add12/1 -> Integrator1/1
  xc1/1 -> Add11/1
  Gain14/1 -> Product14/2
  Gain20/1 -> Add12/2
  Integrator1/1 -> cons1/1, Gain19/1, Add10/2
  Derivative3/1 -> Gain17/1
  Gain16/1 -> Add11/2, Scope/1, alf1/1
  Gain19/1 -> Add12/1
  Add11/1 -> Gain20/1
  PPC/1(z1) -> Gain15/1, To Workspace/1, z1/1, Add10/1
  chiduhanshu/1(Out1) -> Fcn/1, Derivative1/1
  Derivative1/1 -> Abs/1
  Abs/1 -> Product1/1
  Fcn/1 -> Product1/2
  Product1/1 -> Product14/1

== system PPTS_pmsm/uq/alf2 ==
  s2 : Inport
  wm : Inport  Port=2
  z2 : Inport  Port=3
  xc1 : Inport  Port=4
  TL : Inport  Port=5
  d1g : Inport  Port=6
  Abs : Abs
  Add3 : Sum  Inputs=--+++-
  Derivative : Derivative
  Derivative2 : Derivative
  Fcn : Fcn  Expr=1/u
  Gain : Gain  Gain=J/(P*psi_f)
  Gain10 : Gain  Gain=2
  Gain13 : Gain  Gain=1/J
  Gain3 : Gain  Gain=B/J
  Gain6 : Gain  Gain=k2
  Product1 : Product
  Product2 : Product
  chiduhanshu : Subsystem
  alf2 : Outport
  wires:
  Derivative2/1 -> Add3/5
  Add3/1 -> Gain/1
  Gain13/1 -> Add3/4
  Gain3/1 -> Add3/3
  Gain6/1 -> Add3/1
  Product2/1 -> Add3/2
  Gain/1 -> alf2/1
  xc1/1 -> Derivative2/1
  z2/1 -> Gain6/1
  wm/1 -> Gain3/1
  s2/1 -> Gain10/1
  Gain10/1 -> Product2/2
  TL/1 -> Gain13/1
  d1g/1 -> Add3/6
  Product1/1 -> Product2/1
  chiduhanshu/1(Out1) -> Derivative/1, Fcn/1
  Fcn/1 -> Product1/2
  Derivative/1 -> Abs/1
  Abs/1 -> Product1/1

== system PPTS_pmsm/uq/chiduhanshu ==
  Clock : Clock
  Clock1 : Clock
  Constant1 : Constant  Value=T
  Constant{2,4..6} (4 alike) : Constant
  Constant3 : Constant  Value=T
  Constant7 : Constant  Value=T
  Constant8 : Constant  Value=1/T
  Exp : Math  SaturateOnIntegerOverflow=on
  Fcn : Fcn  Expr=u^3
  Gain7 : Gain  Gain=a
  Gain8 : Gain  Gain=a
  Product : Product
  Subtract{1..6} (6 alike) : Sum  Inputs=+-
  Switch : Switch  Threshold=T
  Switch1 : Switch  Threshold=T
  Tanh : Trigonometry  Operator=tanh
  Out1 : Outport
  wires:
  Subtract5/1 -> Switch/3
  Gain7/1 -> Tanh/1
  Subtract4/1 -> Gain8/1
  Gain8/1 -> Exp/1
  Clock/1 -> Subtract4/2, Switch/2, Subtract2/1
  Exp/1 -> Subtract5/1
  Constant1/1 -> Subtract2/2
  Constant2/1 -> Subtract3/1
  Subtract2/1 -> Gain7/1
  Subtract3/1 -> Switch/1
  Tanh/1 -> Subtract3/2
  Constant3/1 -> Subtract4/1
  Constant4/1 -> Subtract5/2
  Constant5/1 -> Switch1/1
  Clock1/1 -> Subtract6/2, Switch1/2
  Constant6/1 -> Subtract1/1
  Constant7/1 -> Subtract6/1
  Subtract6/1 -> Product/1
  Constant8/1 -> Product/2
  Product/1 -> Fcn/1
  Fcn/1 -> Subtract1/2
  Subtract1/1 -> Switch1/3
  Switch/1 -> Out1/1

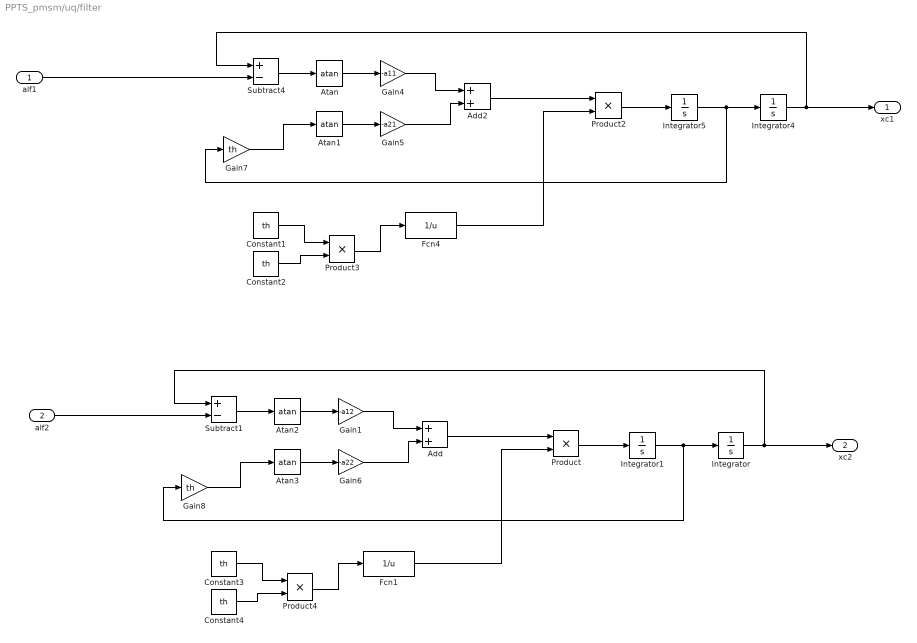
== system PPTS_pmsm/uq/filter ==
  alf1 : Inport
  alf2 : Inport  Port=2
  Add : Sum
  Add2 : Sum
  Atan{,1..3} (4 alike) : Trigonometry  Operator=atan
  Constant{1..4} (4 alike) : Constant  Value=th
  Fcn1 : Fcn  Expr=1/u
  Fcn4 : Fcn  Expr=1/u
  Gain1 : Gain  Gain=-a12
  Gain4 : Gain  Gain=-a11
  Gain5 : Gain  Gain=-a21
  Gain6 : Gain  Gain=-a22
  Gain7 : Gain  Gain=th
  Gain8 : Gain  Gain=th
  Integrator{,1,4..5} (4 alike) : Integrator
  Product{,2..4} (4 alike) : Product
  Subtract1 : Sum  Inputs=+-
  Subtract4 : Sum  Inputs=+-
  xc1 : Outport
  xc2 : Outport  Port=2
  wires:
  Constant2/1 -> Product3/2
  Gain4/1 -> Add2/1
  Gain5/1 -> Add2/2
  Gain7/1 -> Atan1/1
  Product3/1 -> Fcn4/1
  Constant1/1 -> Product3/1
  Integrator5/1 -> Integrator4/1, Gain7/1
  Add2/1 -> Product2/1
  alf1/1 -> Subtract4/2
  Integrator4/1 -> xc1/1, Subtract4/1
  Subtract4/1 -> Atan/1
  Fcn4/1 -> Product2/2
  Atan1/1 -> Gain5/1
  Atan/1 -> Gain4/1
  Product2/1 -> Integrator5/1
  Constant4/1 -> Product4/2
  Gain1/1 -> Add/1
  Gain6/1 -> Add/2
  Gain8/1 -> Atan3/1
  Product4/1 -> Fcn1/1
  Constant3/1 -> Product4/1
  Integrator1/1 -> Integrator/1, Gain8/1
  Add/1 -> Product/1
  alf2/1 -> Subtract1/2
  Integrator/1 -> xc2/1, Subtract1/1
  Subtract1/1 -> Atan2/1
  Fcn1/1 -> Product/2
  Atan3/1 -> Gain6/1
  Atan2/1 -> Gain1/1
  Product/1 -> Integrator1/1

== system PPTS_pmsm/uq2/alf1 ==
  thetad : Inport
  theta-thetad : Inport  Port=2
  Add5 : Sum  Inputs=--+
  Derivative : Derivative
  Gain1 : Gain  Gain=K1
  Gain16 : Gain  Gain=rh0c
  Gain2 : Gain  Gain=1/rh0c
  PPC : Subsystem
  alf1 : Outport
  ppc : Outport  Port=2
  wires:
  Add5/1 -> Gain16/1
  Gain16/1 -> alf1/1
  thetad/1 -> Derivative/1
  Derivative/1 -> Gain2/1
  PPC/2(beta) -> Add5/2
  theta-thetad/1 -> PPC/1(theta-thetad)
  Gain1/1 -> Add5/1
  PPC/1(s1) -> Gain1/1
  Gain2/1 -> Add5/3
  PPC/3(Out1) -> ppc/1

== system PPTS_pmsm/uq2/alf2 ==
  s2 : Inport
  wm : Inport  Port=2
  alf1 : Inport  Port=3
  TL : Inport  Port=4
  Add3 : Sum  Inputs=-++-
  Derivative2 : Derivative
  Gain : Gain  Gain=J/(P*psi_f)
  Gain13 : Gain  Gain=1/J
  Gain2 : Gain  Gain=K2
  Gain3 : Gain  Gain=B/J
  alf2 : Outport
  wires:
  Add3/1 -> Gain/1
  Gain/1 -> alf2/1
  TL/1 -> Gain13/1
  wm/1 -> Gain3/1
  alf1/1 -> Derivative2/1
  Gain13/1 -> Add3/4
  Gain3/1 -> Add3/3
  Derivative2/1 -> Add3/2
  Gain2/1 -> Add3/1
  s2/1 -> Gain2/1

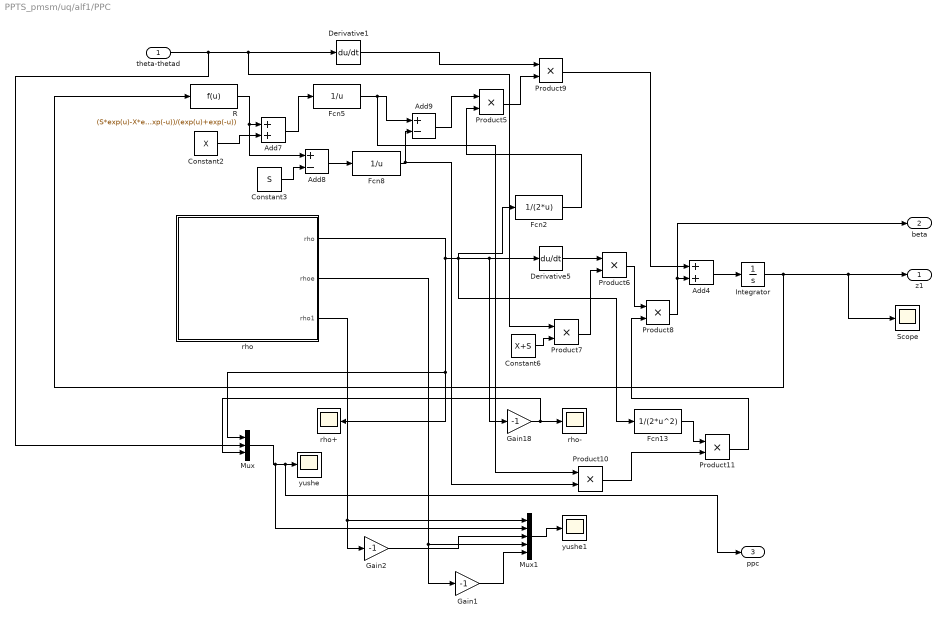
== system PPTS_pmsm/uq/alf1/PPC ==
  theta-thetad : Inport
  Add4 : Sum
  Add7 : Sum
  Add8 : Sum  Inputs=+-
  Add9 : Sum  Inputs=+-
  Constant2 : Constant  Value=X
  Constant3 : Constant  Value=S
  Constant6 : Constant  Value=X+S
  Derivative1 : Derivative
  Derivative5 : Derivative
  Fcn13 : Fcn  Expr=1/(2*u^2)
  Fcn2 : Fcn  Expr=1/(2*u)
  Fcn5 : Fcn  Expr=1/u
  Fcn8 : Fcn  Expr=1/u
  Gain1 : Gain  Gain=-1
  Gain18 : Gain  Gain=-1
  Gain2 : Gain  Gain=-1
  Integrator : Integrator
  Mux : Mux  Inputs=3
  Mux1 : Mux  Inputs=5
  Product{5..11} (7 alike) : Product
  R : Fcn  Expr=(S*exp(u)-X*exp(-u))/(exp(u)+exp(-u))
  Scope : Scope
  rho : Subsystem
  rho+ : Scope
  rho- : Scope
  yushe : Scope
  yushe1 : Scope
  z1 : Outport
  beta : Outport  Port=2
  ppc : Outport  Port=3
  wires:
  theta-thetad/1 -> Mux/2, Product7/1, Derivative1/1
  Product7/1 -> Product6/2
  Fcn13/1 -> Product11/1
  Product9/1 -> Add4/1
  Product8/1 -> beta/1, Add4/2
  Product5/1 -> Product9/2
  Mux/1 -> Mux1/2, ppc/1, yushe/1
  Add4/1 -> Integrator/1
  Derivative1/1 -> Product9/1
  Integrator/1 -> Scope/1, z1/1, R/1
  Fcn8/1 -> Product10/2, Add9/2
  Derivative5/1 -> Product6/1
  Constant3/1 -> Add8/2
  Fcn2/1 -> Product5/2
  Add7/1 -> Fcn5/1
  Fcn5/1 -> Product10/1, Add9/1
  Gain18/1 -> Mux/3, rho-/1
  Add8/1 -> Fcn8/1
  Constant2/1 -> Add7/2
  Product6/1 -> Product8/1
  R/1 -> Add8/1, Add7/1
  Add9/1 -> Product5/1
  Product11/1 -> Product8/2
  Constant6/1 -> Product7/2
  Product10/1 -> Product11/2
  rho/1(rho) -> Mux/1, rho+/1, Fcn13/1, Gain18/1, Derivative5/1, Fcn2/1
  Mux1/1 -> yushe1/1
  rho/3(rho1) -> Gain2/1, Mux1/1
  Gain2/1 -> Mux1/3
  rho/2(rhoe) -> Gain1/1, Mux1/4
  Gain1/1 -> Mux1/5

== system PPTS_pmsm/uq/alf1/chiduhanshu ==
  Clock : Clock
  Clock1 : Clock
  Constant1 : Constant  Value=T
  Constant{2,4..6} (4 alike) : Constant
  Constant3 : Constant  Value=T
  Constant7 : Constant  Value=T
  Constant8 : Constant  Value=1/T
  Exp : Math  SaturateOnIntegerOverflow=on
  Fcn : Fcn  Expr=u^3
  Gain7 : Gain  Gain=a
  Gain8 : Gain  Gain=a
  Product : Product
  Subtract{1..6} (6 alike) : Sum  Inputs=+-
  Switch : Switch  Threshold=T
  Switch1 : Switch  Threshold=T
  Tanh : Trigonometry  Operator=tanh
  Out1 : Outport
  wires:
  Subtract5/1 -> Switch/3
  Gain7/1 -> Tanh/1
  Subtract4/1 -> Gain8/1
  Gain8/1 -> Exp/1
  Clock/1 -> Subtract4/2, Switch/2, Subtract2/1
  Exp/1 -> Subtract5/1
  Constant1/1 -> Subtract2/2
  Constant2/1 -> Subtract3/1
  Subtract2/1 -> Gain7/1
  Subtract3/1 -> Switch/1
  Tanh/1 -> Subtract3/2
  Constant3/1 -> Subtract4/1
  Constant4/1 -> Subtract5/2
  Constant5/1 -> Switch1/1
  Clock1/1 -> Subtract6/2, Switch1/2
  Constant6/1 -> Subtract1/1
  Constant7/1 -> Subtract6/1
  Subtract6/1 -> Product/1
  Constant8/1 -> Product/2
  Product/1 -> Fcn/1
  Fcn/1 -> Subtract1/2
  Subtract1/1 -> Switch1/3
  Switch/1 -> Out1/1

== system PPTS_pmsm/uq/alf2/chiduhanshu ==
  Clock : Clock
  Clock1 : Clock
  Constant1 : Constant  Value=T
  Constant{2,4..6} (4 alike) : Constant
  Constant3 : Constant  Value=T
  Constant7 : Constant  Value=T
  Constant8 : Constant  Value=1/T
  Exp : Math  SaturateOnIntegerOverflow=on
  Fcn : Fcn  Expr=u^3
  Gain7 : Gain  Gain=a
  Gain8 : Gain  Gain=a
  Product : Product
  Subtract{1..6} (6 alike) : Sum  Inputs=+-
  Switch : Switch  Threshold=T
  Switch1 : Switch  Threshold=T
  Tanh : Trigonometry  Operator=tanh
  Out1 : Outport
  wires:
  Subtract5/1 -> Switch/3
  Gain7/1 -> Tanh/1
  Subtract4/1 -> Gain8/1
  Gain8/1 -> Exp/1
  Clock/1 -> Subtract4/2, Switch/2, Subtract2/1
  Exp/1 -> Subtract5/1
  Constant1/1 -> Subtract2/2
  Constant2/1 -> Subtract3/1
  Subtract2/1 -> Gain7/1
  Subtract3/1 -> Switch/1
  Tanh/1 -> Subtract3/2
  Constant3/1 -> Subtract4/1
  Constant4/1 -> Subtract5/2
  Constant5/1 -> Switch1/1
  Clock1/1 -> Subtract6/2, Switch1/2
  Constant6/1 -> Subtract1/1
  Constant7/1 -> Subtract6/1
  Subtract6/1 -> Product/1
  Constant8/1 -> Product/2
  Product/1 -> Fcn/1
  Fcn/1 -> Subtract1/2
  Subtract1/1 -> Switch1/3
  Switch/1 -> Out1/1

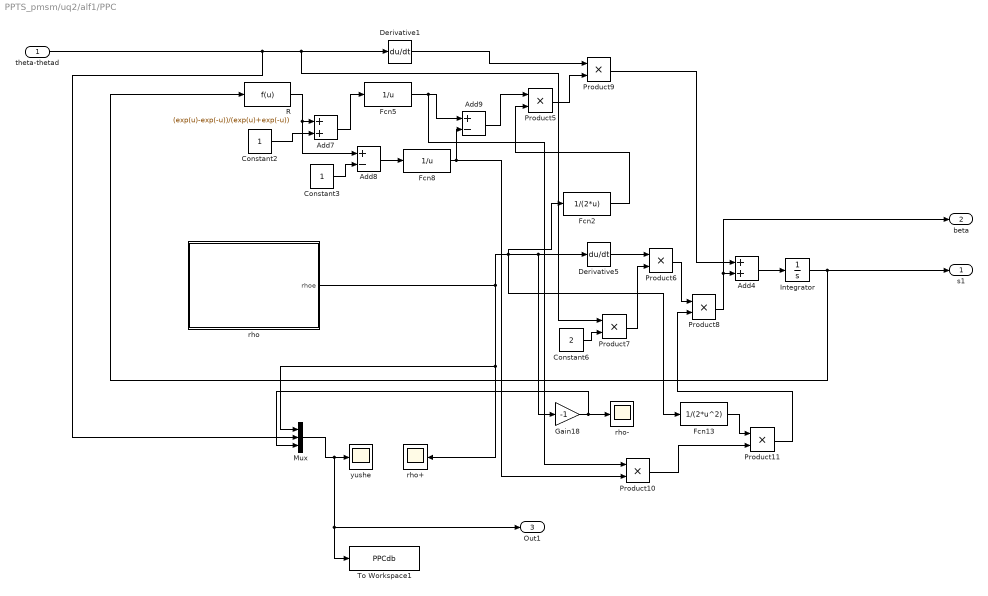
== system PPTS_pmsm/uq2/alf1/PPC ==
  theta-thetad : Inport
  Add4 : Sum
  Add7 : Sum
  Add8 : Sum  Inputs=+-
  Add9 : Sum  Inputs=+-
  Constant2 : Constant
  Constant3 : Constant
  Constant6 : Constant  Value=2
  Derivative1 : Derivative
  Derivative5 : Derivative
  Fcn13 : Fcn  Expr=1/(2*u^2)
  Fcn2 : Fcn  Expr=1/(2*u)
  Fcn5 : Fcn  Expr=1/u
  Fcn8 : Fcn  Expr=1/u
  Gain18 : Gain  Gain=-1
  Integrator : Integrator
  Mux : Mux  Inputs=3
  Product{5..11} (7 alike) : Product
  R : Fcn  Expr=(exp(u)-exp(-u))/(exp(u)+exp(-u))
  To Workspace1 : ToWorkspace  VariableName=PPCdb  SaveFormat=Timeseries  SampleTime=-1
  rho : Subsystem
  rho+ : Scope
  rho- : Scope
  yushe : Scope
  s1 : Outport
  beta : Outport  Port=2
  Out1 : Outport  Port=3
  wires:
  theta-thetad/1 -> Mux/2, Product7/1, Derivative1/1
  Product7/1 -> Product6/2
  Fcn13/1 -> Product11/1
  Product9/1 -> Add4/1
  Product8/1 -> beta/1, Add4/2
  Product5/1 -> Product9/2
  Mux/1 -> To Workspace1/1, Out1/1, yushe/1
  Add4/1 -> Integrator/1
  Derivative1/1 -> Product9/1
  Integrator/1 -> s1/1, R/1
  Fcn8/1 -> Product10/2, Add9/2
  Derivative5/1 -> Product6/1
  Constant3/1 -> Add8/2
  Fcn2/1 -> Product5/2
  Add7/1 -> Fcn5/1
  Fcn5/1 -> Product10/1, Add9/1
  Gain18/1 -> Mux/3, rho-/1
  Add8/1 -> Fcn8/1
  Constant2/1 -> Add7/2
  Product6/1 -> Product8/1
  R/1 -> Add8/1, Add7/1
  Add9/1 -> Product5/1
  Product11/1 -> Product8/2
  Constant6/1 -> Product7/2
  Product10/1 -> Product11/2
  rho/1(rhoe) -> Fcn13/1, Gain18/1, Derivative5/1, Fcn2/1, Mux/1, rho+/1

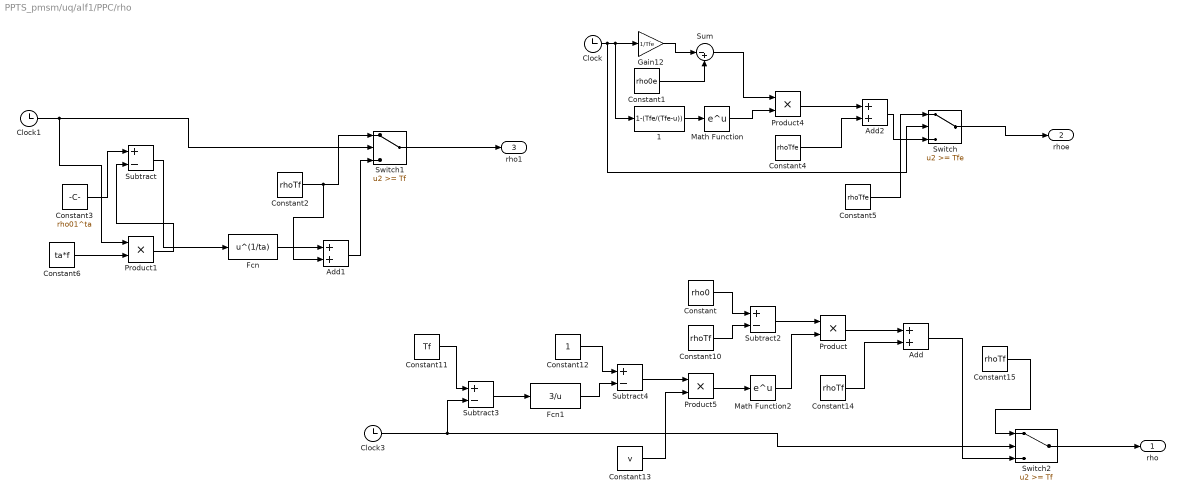
== system PPTS_pmsm/uq/alf1/PPC/rho ==
  1 : Fcn  Expr=1-(Tfe/(Tfe-u))
  Add : Sum
  Add1 : Sum
  Add2 : Sum
  Clock : Clock
  Clock1 : Clock
  Clock3 : Clock
  Constant : Constant  Value=rho0
  Constant1 : Constant  Value=rho0e
  Constant{2,10,14..15} (4 alike) : Constant  Value=rhoTf
  Constant11 : Constant  Value=Tf
  Constant12 : Constant
  Constant13 : Constant  Value=v
  Constant3 : Constant  Value=rho01^ta
  Constant4 : Constant  Value=rhoTfe
  Constant5 : Constant  Value=rhoTfe
  Constant6 : Constant  Value=ta*f
  Fcn : Fcn  Expr=u^(1/ta)
  Fcn1 : Fcn  Expr=3/u
  Gain12 : Gain  Gain=1/Tfe
  Math Function : Math  SaturateOnIntegerOverflow=on
  Math Function2 : Math  SaturateOnIntegerOverflow=on
  Product{,1,4..5} (4 alike) : Product
  Subtract{,2..4} (4 alike) : Sum  Inputs=+-
  Sum : Sum  Inputs=|-+
  Switch : Switch  Threshold=Tfe
  Switch1 : Switch  Threshold=Tf
  Switch2 : Switch  Threshold=Tf
  rho : Outport
  rhoe : Outport  Port=2
  rho1 : Outport  Port=3
  wires:
  Gain12/1 -> Sum/1
  Sum/1 -> Product4/1
  Clock/1 -> Switch/2, 1/1, Gain12/1
  Math Function/1 -> Product4/2
  Add2/1 -> Switch/3
  Constant4/1 -> Add2/2
  1/1 -> Math Function/1
  Constant1/1 -> Sum/2
  Product4/1 -> Add2/1
  Constant5/1 -> Switch/1
  Switch2/1 -> rho/1
  Switch/1 -> rhoe/1
  Fcn1/1 -> Subtract4/2
  Math Function2/1 -> Product/2
  Subtract3/1 -> Fcn1/1
  Constant13/1 -> Product5/2
  Constant12/1 -> Subtract4/1
  Constant10/1 -> Subtract2/2
  Product/1 -> Add/1
  Product5/1 -> Math Function2/1
  Constant/1 -> Subtract2/1
  Clock3/1 -> Switch2/2, Subtract3/2
  Constant11/1 -> Subtract3/1
  Subtract4/1 -> Product5/1
  Constant15/1 -> Switch2/1
  Add/1 -> Switch2/3
  Subtract2/1 -> Product/1
  Constant14/1 -> Add/2
  Switch1/1 -> rho1/1
  Subtract/1 -> Fcn/1
  Add1/1 -> Switch1/3
  Fcn/1 -> Add1/1
  Product1/1 -> Subtract/2
  Constant3/1 -> Subtract/1
  Constant6/1 -> Product1/2
  Clock1/1 -> Product1/1, Switch1/2
  Constant2/1 -> Add1/2, Switch1/1

== system PPTS_pmsm/uq2/alf1/PPC/rho ==
  1 : Fcn  Expr=1-(Tfc/(Tfc-u))
  Add2 : Sum
  Clock : Clock
  Constant1 : Constant  Value=rho0c
  Constant4 : Constant  Value=rhoTfc
  Constant5 : Constant  Value=rhoTfc
  Gain12 : Gain  Gain=1/Tfc
  Math Function : Math  SaturateOnIntegerOverflow=on
  Product4 : Product
  Sum : Sum  Inputs=|-+
  Switch : Switch  Threshold=Tfc
  rhoe : Outport
  wires:
  Gain12/1 -> Sum/1
  Sum/1 -> Product4/1
  Clock/1 -> Switch/2, 1/1, Gain12/1
  Math Function/1 -> Product4/2
  Add2/1 -> Switch/3
  Constant4/1 -> Add2/2
  1/1 -> Math Function/1
  Constant1/1 -> Sum/2
  Product4/1 -> Add2/1
  Constant5/1 -> Switch/1
  Switch/1 -> rhoe/1

== matlab function PPTS_pmsm/pmsm/MATLAB Function1 ==
  data: u1 input; y output; u2 input
function y = fcn(u1,u2)
if u1<0.2
    y=0;
elseif u1>=2
        y=(1/u2)*0.5*sin(2*pi*u1);
else
     y=(1/u2)*2.8*sin(0.25*u1);
end

== matlab function PPTS_pmsm/pmsm/MATLAB Function ==
  data: u1 input; y output; u2 input; u3 input
function y = fcn(u1,u2,u3)
if u1<0.2
    y=0;
elseif u1>=2
            y=u3-1;
else
    y=u2-1
end
